simulink model "Task_space"  (R2023a)
settings: Solver=VariableStepAuto  StartTime=0.0  StopTime=10  RelTol=1e-3
undefined symbols (not defined in the file or in its folder): smiData, smiData1, X, Y, Z
libraries: sm_lib x270, nesl_utility x32, simulink_extras x8
(part 6 of 6)

== matlab function Task_space/MATLAB Function1 ==
  data: q input; X output
function X = arm_forward_kinematics(q)
q1 = q(1);
q2 = q(2);
q3 = q(3);
q4 = q(4);
l1 = 0.02888;
l2 = 0.02659;
l3 = 0.1224;
l4 = 0.15;

X = [l4*cos((pi*q1)/180)*sin((pi*(q2-90))/180)*sin((pi*(q4-90))/180)-l4*cos((pi*(q4-90))/180)*(sin((pi*q1)/180)*sin((pi*(q3-90))/180)-cos((pi*q1)/180)*cos((pi*(q2-90))/180)*cos((pi*(q3-90))/180))-cos((pi*q1)/180)*sin((pi*(q2-90))/180)*(l2+l3);
    l4*cos((pi*(q4-90))/180)*(cos((pi*q1)/180)*sin((pi*(q3-90))/180)+sin((pi*q1)/180)*cos((pi*(q2-90))/180)*cos((pi*(q3-90))/180))-sin((pi*q1)/180)*sin((pi*(q2-90))/180)*(l2+l3)+l4*sin((pi*q1)/180)*sin((pi*(q2-90))/180)*sin((pi*(q4-90))/180);
    l4*cos((pi*(q2-90))/180)*sin((pi*(q4-90))/180)-cos((pi*(q2-90))/180)*(l2+l3)-l1-l4*cos((pi*(q3-90))/180)*cos((pi*(q4-90))/180)*sin((pi*(q2-90))/180)];
      
x = X(1,1);
y = X(2,1);
z = X(3,1);
X = [x;y;z]
